simulink model "Threephaseplll"  (R2015b)
settings: Solver=VariableStepAuto  StartTime=0.0  StopTime=0.5  RelTol=1e-3
undefined symbols (not defined in the file): c, k, n, Ts, w1
libraries: powerlib_meascontrol x1, simulink x1, powerlib x1
settings Model: Creator=HP  LastModifiedBy=HP

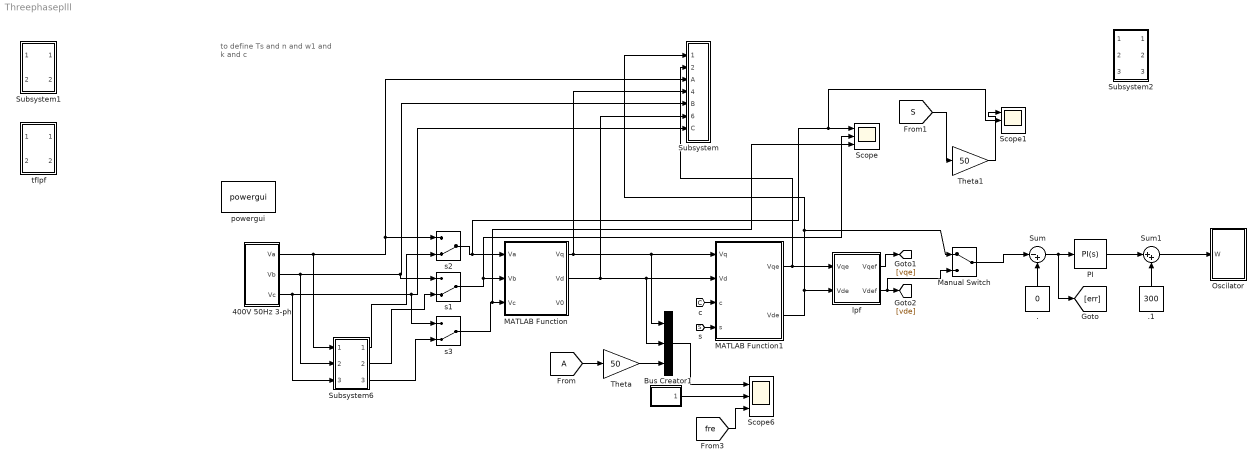
== system Threephaseplll ==
  note: to define Ts  and n
      | and w1 and k and c
  "               " : Subsystem
  . : Constant  Value=0
  .1 : Constant  Value=300
  400V 50Hz 3-ph : Subsystem
  Bus Creator1 : BusCreator  Inputs=3
  MATLAB Function : MATLAB Function  TreatAsAtomicUnit=on
  MATLAB Function1 : MATLAB Function  TreatAsAtomicUnit=on
  Manual Switch : ManualSwitch
  Oscilator : Subsystem
  PI : simulink/Continuous/PID Controller  Controller=PI  TimeDomain=Continuous-time  SampleTime=-1  IntegratorMethod=Forward Euler  FilterMethod=Forward Euler  Form=Parallel  UseFilter=on  ControllerParametersSource=internal  P=4  I=30  D=0  N=100  InitialConditionSource=internal  InitialConditionForIntegrator=0  InitialConditionForFilter=0  ExternalReset=none  ZeroCross=off  LimitOutput=off  UpperSaturationLimit=inf  LowerSaturationLimit=-inf  LinearizeAsGain=on  AntiWindupMode=none  Kb=1  TrackingMode=off  Kt=1  PParamMin=[]  PParamMax=[]  IParamMin=[]  IParamMax=[]  DParamMin=[]  DParamMax=[]  NParamMin=[]  NParamMax=[]  KbParamMin=[]  KbParamMax=[]  KtParamMin=[]  KtParamMax=[]  POutMin=[]  POutMax=[]  IOutMin=[]  IOutMax=[]  DOutMin=[]  DOutMax=[]  NOutMin=[]  NOutMax=[]  KbOutMin=[]  KbOutMax=[]  KtOutMin=[]  KtOutMax=[]  IntegratorOutMin=[]  IntegratorOutMax=[]  FilterOutMin=[]  FilterOutMax=[]  SumOutMin=[]  SumOutMax=[]  SumI1OutMin=[]  SumI1OutMax=[]  SumI2OutMin=[]  SumI2OutMax=[]  SumI3OutMin=[]  SumI3OutMax=[]  SumDOutMin=[]  SumDOutMax=[]  SaturationOutMin=[]  SaturationOutMax=[]  IntegratorContinuousStateAttributes=''  IntegratorStateMustResolveToSignalObject=off  IntegratorRTWStateStorageClass=Auto  FilterContinuousStateAttributes=''  FilterStateMustResolveToSignalObject=off  FilterRTWStateStorageClass=Auto  DifferentiatorICPrevScaledInput=0  DifferentiatorOutMin=[]  DifferentiatorOutMax=[]
  Scope : Scope  NumInputPorts=3
  Scope1 : Scope  NumInputPorts=3
  Scope6 : Scope  NumInputPorts=3
  Subsystem : Subsystem
  Subsystem1 : Subsystem
  Subsystem2 : Subsystem
  Subsystem6 : Subsystem
  Sum : Sum  Inputs=|-+
  Sum1 : Sum  Inputs=|++
  Theta : Gain  Gain=50
  Theta1 : Gain  Gain=50
  lpf : Subsystem
  powergui : powerlib/powergui  Priority=1  SimulationMode=Discrete  SolverType=Tustin/Backward Euler (TBE)  SampleTime=50e-6  frequency=60  SPID=on  DisableSnubberDevices=off  DisableRonSwitches=off  DisableVfSwitches=off  SwTol=0  DisplayEquations=on  Interpol=off  ExternalGateDelay=off  methode=off  Ts=10  FunctionMessages=off  echomessages=off  HookPort=off  EnableUseOfTLC=off  x0status=blocks  frequencyindice=50  Pbase=100e6  ErrMax=1e-4  Iterations=50  UnitsV=kV  UnitsW=MW  buscounter=0  RestoreLinks=warning  ResistiveCurrentMeasurement=off  Frange=[0:2:500]  Ylog=off  Xlog=on  ShowGrid=off  save=off  variable=ZData  structure=Vload  ZoomFFT=on  StartTime=0.2  cycles=4  DisplayStyle=3  fundamental=50  FreqAxis=on  MaxFrequency=1000  frequencyindicesteady=1  RmsSteady=1  display=off
  s1 : ManualSwitch  CurrentSetting=0
  s2 : ManualSwitch  CurrentSetting=0
  "s3 " : ManualSwitch  CurrentSetting=0
  tflpf : Subsystem
  wires:
  400V 50Hz 3-ph/1(Va) -> s2/1, Subsystem/3(A), Subsystem6/1(In1)
  400V 50Hz 3-ph/2(Vb) -> s1/1, Subsystem/5(B), Subsystem6/2(In2)
  400V 50Hz 3-ph/3(Vc) -> "s3 "/1, Subsystem/7(C), Subsystem6/3(In3)
  MATLAB Function/2(Vd) -> Subsystem/6("Vd "), MATLAB Function1/2(Vd), Bus Creator1/2
  Sum/1 -> [err], PI/1
  .1/1 -> Sum1/2
  MATLAB Function1/2(Vde) -> Manual Switch/1, Subsystem/1(Vde), lpf/2(Vde)
  ./1 -> Sum/2
  MATLAB Function/1(Vq) -> Subsystem/4(Vq), MATLAB Function1/1(Vq), Bus Creator1/1
  PI/1 -> Sum1/1
  MATLAB Function1/1(Vqe) -> Subsystem/2(Vqe), lpf/1(Vqe)
  Manual Switch/1 -> Sum/1
  lpf/2(Vdef) -> Manual Switch/2, [vde]
  [S] -> MATLAB Function1/4(s)
  [C] -> MATLAB Function1/3(c)
  lpf/1(Vqef) -> [vqe]
  Sum1/1 -> Oscilator/1(W)
  Theta/1 -> Bus Creator1/3
  [fre] -> Scope6/3
  Bus Creator1/1 -> Scope6/1
  [A] -> Theta/1
  "               "/1(Error PI) -> Scope6/2
  s2/1 -> Scope1/2, Scope/1, MATLAB Function/1(Va)
  s1/1 -> Scope/2, MATLAB Function/2(Vb)
  "s3 "/1 -> Scope/3, MATLAB Function/3(Vc)
  Subsystem6/1(Out1) -> s2/2
  Subsystem6/2(Out2) -> s1/2
  Subsystem6/3(Out3) -> "s3 "/2
  [S] -> Theta1/1
  Theta1/1 -> Scope1/1

== system Threephaseplll/                ==
  Error : Gain
  Error PI : Outport
  wires:
  Error/1 -> Error PI/1
  [err] -> Error/1

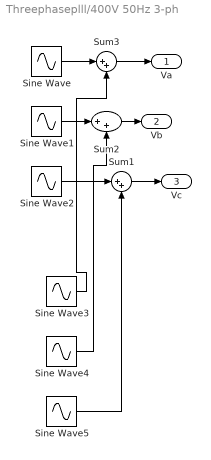
== system Threephaseplll/400V 50Hz 3-ph ==
  Sine Wave : Sin  Amplitude=c*400*sqrt(2)/sqrt(3)  Frequency=w1  SampleTime=Ts
  Sine Wave1 : Sin  Amplitude=400*sqrt(2)/sqrt(3)  Frequency=w1  Phase=-2*pi/3  SampleTime=Ts
  Sine Wave2 : Sin  Amplitude=400*sqrt(2)/sqrt(3)  Frequency=w1  Phase=-4*pi/3  SampleTime=Ts
  Sine Wave3 : Sin  Amplitude=0.2*400*sqrt(2)/sqrt(3)*k  Frequency=w1*n  SampleTime=Ts
  Sine Wave4 : Sin  Amplitude=0.2*k*400*sqrt(2)/sqrt(3)  Frequency=w1*n  Phase=-2*pi/3*n  SampleTime=Ts
  Sine Wave5 : Sin  Amplitude=0.2*k*400*sqrt(2)/sqrt(3)  Frequency=w1*n  Phase=-4*pi/3*n  SampleTime=Ts
  Sum1 : Sum  Inputs=|++
  Sum2 : Sum  Inputs=|++
  Sum3 : Sum  Inputs=|++
  Va : Outport
  Vb : Outport  Port=2
  Vc : Outport  Port=3
  wires:
  Sine Wave/1 -> Sum3/1
  Sum3/1 -> Va/1
  Sine Wave1/1 -> Sum2/1
  Sum2/1 -> Vb/1
  Sine Wave2/1 -> Sum1/1
  Sum1/1 -> Vc/1
  Sine Wave3/1 -> Sum3/2
  Sine Wave4/1 -> Sum2/2
  Sine Wave5/1 -> Sum1/2

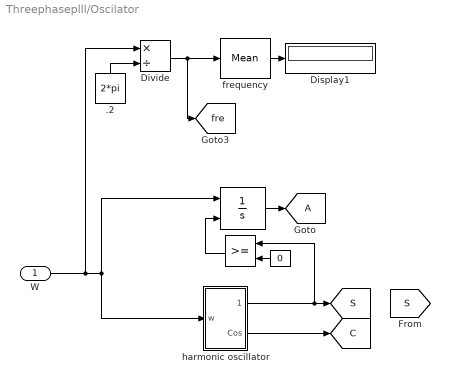
== system Threephaseplll/Oscilator ==
  W : Inport
  " " : Constant  Value=0
  "  " : Integrator  ExternalReset=rising  UpperSaturationLimit=2*pi  LowerSaturationLimit=0
  "    " : RelationalOperator  OutDataTypeStr=boolean
  .2 : Constant  Value=2*pi
  Display1 : Display
  Divide : Product  Inputs=*/
  frequency : powerlib_meascontrol/Measurements/Mean  Freq=60  Vinit=0  Ts=0
  "harmonic oscillator " : Subsystem
  tag scope: A=global, C=global, S=global, fre=global
  wires:
  .2/1 -> Divide/2
  "harmonic oscillator "/1(Sine) -> "    "/1, [S]
  "  "/1 -> [A]
  " "/1 -> "    "/2
  W/1 -> "harmonic oscillator "/1(w), "  "/1, Divide/1
  "    "/1 -> "  "/2
  frequency/1 -> Display1/1
  Divide/1 -> [fre], frequency/1
  "harmonic oscillator "/2(Cos) -> [C]

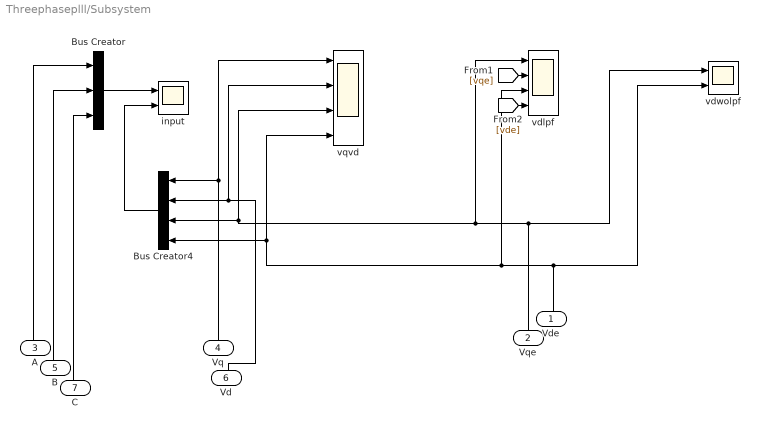
== system Threephaseplll/Subsystem ==
  Vde : Inport
  Vqe : Inport  Port=2
  A : Inport  Port=3
  Vq : Inport  Port=4
  B : Inport  Port=5
  "Vd " : Inport  Port=6
  C : Inport  Port=7
  Bus Creator : BusCreator  Inputs=3
  Bus Creator4 : BusCreator  Inputs=4
  input : Scope  NumInputPorts=2
  vdlpf : Scope  NumInputPorts=4
  vdwolpf : Scope  NumInputPorts=2
  vqvd : Scope  NumInputPorts=4
  wires:
  [vqe] -> vdlpf/2
  Bus Creator/1 -> input/1
  Bus Creator4/1 -> input/2
  "Vd "/1 -> vqvd/2, Bus Creator4/2
  A/1 -> Bus Creator/1
  B/1 -> Bus Creator/2
  Vq/1 -> vqvd/1, Bus Creator4/1
  Vqe/1 -> vdwolpf/1, vdlpf/1, vqvd/3, Bus Creator4/3
  C/1 -> Bus Creator/3
  Vde/1 -> vdwolpf/2, vdlpf/3, vqvd/4, Bus Creator4/4
  [vde] -> vdlpf/4

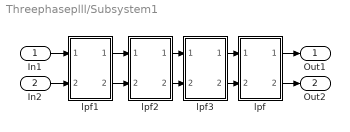
== system Threephaseplll/Subsystem1 ==
  In1 : Inport
  In2 : Inport  Port=2
  lpf : Subsystem
  lpf1 : Subsystem
  lpf2 : Subsystem
  lpf3 : Subsystem
  Out1 : Outport
  Out2 : Outport  Port=2
  wires:
  lpf1/2(Out2) -> lpf2/2(In2)
  lpf1/1(Out1) -> lpf2/1(In1)
  lpf2/2(Out2) -> lpf3/2(In2)
  lpf2/1(Out1) -> lpf3/1(In1)
  lpf3/1(Out1) -> lpf/1(In1)
  lpf3/2(Out2) -> lpf/2(In2)
  lpf/1(Out1) -> Out1/1
  lpf/2(Out2) -> Out2/1
  In2/1 -> lpf1/2(In2)
  In1/1 -> lpf1/1(In1)

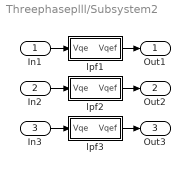
== system Threephaseplll/Subsystem2 ==
  In1 : Inport
  In2 : Inport  Port=2
  In3 : Inport  Port=3
  lpf1 : Subsystem
  lpf2 : Subsystem
  lpf3 : Subsystem
  Out1 : Outport
  Out2 : Outport  Port=2
  Out3 : Outport  Port=3
  wires:
  In2/1 -> lpf2/1(Vqe)
  In3/1 -> lpf3/1(Vqe)
  lpf2/1(Vqef) -> Out2/1
  lpf3/1(Vqef) -> Out3/1
  lpf1/1(Vqef) -> Out1/1
  In1/1 -> lpf1/1(Vqe)

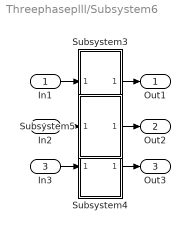
== system Threephaseplll/Subsystem6 ==
  In1 : Inport
  In2 : Inport  Port=2
  In3 : Inport  Port=3
  Subsystem3 : Subsystem
  Subsystem4 : Subsystem
  Subsystem5 : Subsystem
  Out1 : Outport
  Out2 : Outport  Port=2
  Out3 : Outport  Port=3
  wires:
  Subsystem5/1(Out1) -> Out2/1
  In1/1 -> Subsystem3/1(In1)
  Subsystem3/1(Out1) -> Out1/1
  Subsystem4/1(Out1) -> Out3/1
  In2/1 -> Subsystem5/1(In1)
  In3/1 -> Subsystem4/1(In1)

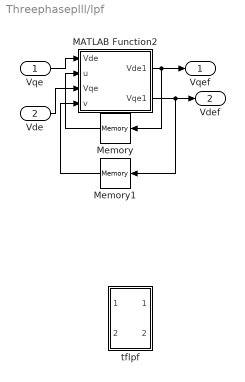
== system Threephaseplll/lpf ==
  Vqe : Inport
  Vde : Inport  Port=2
  MATLAB Function2 : MATLAB Function  TreatAsAtomicUnit=on
  Memory : Memory
  Memory1 : Memory
  tflpf : Subsystem
  Vqef : Outport
  Vdef : Outport  Port=2
  wires:
  MATLAB Function2/1(Vde1) -> Vqef/1, Memory/1
  Vqe/1 -> MATLAB Function2/1(Vde)
  Memory/1 -> MATLAB Function2/2(u)
  Vde/1 -> MATLAB Function2/3(Vqe)
  MATLAB Function2/2(Vqe1) -> Vdef/1, Memory1/1
  Memory1/1 -> MATLAB Function2/4(v)

== system Threephaseplll/tflpf ==
  In1 : Inport
  In2 : Inport  Port=2
  Transfer Fcn : TransferFcn  Numerator=[2*pi*10]  Denominator=[1 2*pi*10]
  Transfer Fcn1 : TransferFcn  Numerator=[2*pi*10]  Denominator=[1 2*pi*10]
  Out1 : Outport
  Out2 : Outport  Port=2
  wires:
  In2/1 -> Transfer Fcn1/1
  In1/1 -> Transfer Fcn/1
  Transfer Fcn/1 -> Out1/1
  Transfer Fcn1/1 -> Out2/1

== system Threephaseplll/Oscilator/harmonic oscillator  ==
  w : Inport
  MATLAB Function2 : MATLAB Function  TreatAsAtomicUnit=on
  Memory : Memory  X0=1
  Memory1 : Memory
  Sine : Outport
  Cos : Outport  Port=2
  wires:
  Memory1/1 -> MATLAB Function2/2(s)
  MATLAB Function2/2(s1) -> Sine/1, Memory1/1
  MATLAB Function2/1(c1) -> Cos/1, Memory/1
  Memory/1 -> MATLAB Function2/3(c)
  w/1 -> MATLAB Function2/1(u)

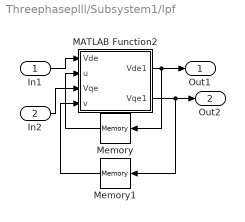
== system Threephaseplll/Subsystem1/lpf ==
  In1 : Inport
  In2 : Inport  Port=2
  MATLAB Function2 : MATLAB Function  TreatAsAtomicUnit=on
  Memory : Memory
  Memory1 : Memory
  Out1 : Outport
  Out2 : Outport  Port=2
  wires:
  MATLAB Function2/1(Vde1) -> Out1/1, Memory/1
  In1/1 -> MATLAB Function2/1(Vde)
  Memory/1 -> MATLAB Function2/2(u)
  In2/1 -> MATLAB Function2/3(Vqe)
  MATLAB Function2/2(Vqe1) -> Out2/1, Memory1/1
  Memory1/1 -> MATLAB Function2/4(v)

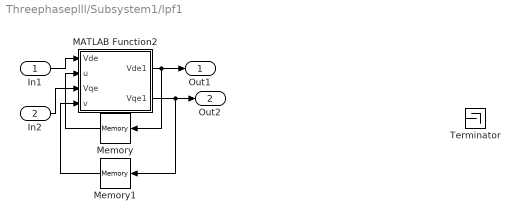
== system Threephaseplll/Subsystem1/lpf1 ==
  In1 : Inport
  In2 : Inport  Port=2
  MATLAB Function2 : MATLAB Function  TreatAsAtomicUnit=on
  Memory : Memory
  Memory1 : Memory
  Terminator : Terminator
  Out1 : Outport
  Out2 : Outport  Port=2
  wires:
  MATLAB Function2/1(Vde1) -> Out1/1, Memory/1
  In1/1 -> MATLAB Function2/1(Vde)
  Memory/1 -> MATLAB Function2/2(u)
  In2/1 -> MATLAB Function2/3(Vqe)
  MATLAB Function2/2(Vqe1) -> Out2/1, Memory1/1
  Memory1/1 -> MATLAB Function2/4(v)

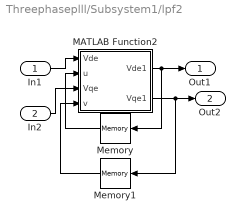
== system Threephaseplll/Subsystem1/lpf2 ==
  In1 : Inport
  In2 : Inport  Port=2
  MATLAB Function2 : MATLAB Function  TreatAsAtomicUnit=on
  Memory : Memory
  Memory1 : Memory
  Out1 : Outport
  Out2 : Outport  Port=2
  wires:
  MATLAB Function2/1(Vde1) -> Out1/1, Memory/1
  In1/1 -> MATLAB Function2/1(Vde)
  Memory/1 -> MATLAB Function2/2(u)
  In2/1 -> MATLAB Function2/3(Vqe)
  MATLAB Function2/2(Vqe1) -> Out2/1, Memory1/1
  Memory1/1 -> MATLAB Function2/4(v)

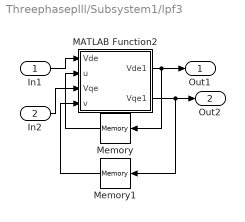
== system Threephaseplll/Subsystem1/lpf3 ==
  In1 : Inport
  In2 : Inport  Port=2
  MATLAB Function2 : MATLAB Function  TreatAsAtomicUnit=on
  Memory : Memory
  Memory1 : Memory
  Out1 : Outport
  Out2 : Outport  Port=2
  wires:
  MATLAB Function2/1(Vde1) -> Out1/1, Memory/1
  In1/1 -> MATLAB Function2/1(Vde)
  Memory/1 -> MATLAB Function2/2(u)
  In2/1 -> MATLAB Function2/3(Vqe)
  MATLAB Function2/2(Vqe1) -> Out2/1, Memory1/1
  Memory1/1 -> MATLAB Function2/4(v)

== system Threephaseplll/Subsystem2/lpf1 ==
  Vqe : Inport
  MATLAB Function2 : MATLAB Function  TreatAsAtomicUnit=on
  Memory : Memory
  Memory1 : Memory
  Vqef : Outport
  wires:
  MATLAB Function2/1(Vde1) -> Vqef/1, Memory/1
  Vqe/1 -> MATLAB Function2/1(Vde)
  Memory/1 -> MATLAB Function2/2(u)
  ? -> MATLAB Function2/3(Vqe)
  MATLAB Function2/2(Vqe1) -> Memory1/1
  Memory1/1 -> MATLAB Function2/4(v)

== system Threephaseplll/Subsystem2/lpf2 ==
  Vqe : Inport
  MATLAB Function2 : MATLAB Function  TreatAsAtomicUnit=on
  Memory : Memory
  Memory1 : Memory
  Vqef : Outport
  wires:
  MATLAB Function2/1(Vde1) -> Vqef/1, Memory/1
  Vqe/1 -> MATLAB Function2/1(Vde)
  Memory/1 -> MATLAB Function2/2(u)
  ? -> MATLAB Function2/3(Vqe)
  MATLAB Function2/2(Vqe1) -> Memory1/1
  Memory1/1 -> MATLAB Function2/4(v)

== system Threephaseplll/Subsystem2/lpf3 ==
  Vqe : Inport
  MATLAB Function2 : MATLAB Function  TreatAsAtomicUnit=on
  Memory : Memory
  Memory1 : Memory
  Vqef : Outport
  wires:
  MATLAB Function2/1(Vde1) -> Vqef/1, Memory/1
  Vqe/1 -> MATLAB Function2/1(Vde)
  Memory/1 -> MATLAB Function2/2(u)
  ? -> MATLAB Function2/3(Vqe)
  MATLAB Function2/2(Vqe1) -> Memory1/1
  Memory1/1 -> MATLAB Function2/4(v)

== system Threephaseplll/Subsystem6/Subsystem3 ==
  In1 : Inport
  Transfer Fcn{,1..3} (4 alike) : TransferFcn  Denominator=[(1/(2*pi*60)) 1]
  Out1 : Outport
  wires:
  Transfer Fcn1/1 -> Out1/1
  In1/1 -> Transfer Fcn/1
  Transfer Fcn3/1 -> Transfer Fcn1/1
  Transfer Fcn/1 -> Transfer Fcn2/1
  Transfer Fcn2/1 -> Transfer Fcn3/1

== system Threephaseplll/Subsystem6/Subsystem4 ==
  In1 : Inport
  Transfer Fcn{,1..3} (4 alike) : TransferFcn  Denominator=[(1/(2*pi*60)) 1]
  Out1 : Outport
  wires:
  Transfer Fcn1/1 -> Out1/1
  In1/1 -> Transfer Fcn/1
  Transfer Fcn3/1 -> Transfer Fcn1/1
  Transfer Fcn/1 -> Transfer Fcn2/1
  Transfer Fcn2/1 -> Transfer Fcn3/1

== system Threephaseplll/Subsystem6/Subsystem5 ==
  In1 : Inport
  Transfer Fcn{,1..3} (4 alike) : TransferFcn  Denominator=[(1/(2*pi*60)) 1]
  Out1 : Outport
  wires:
  Transfer Fcn1/1 -> Out1/1
  In1/1 -> Transfer Fcn/1
  Transfer Fcn3/1 -> Transfer Fcn1/1
  Transfer Fcn/1 -> Transfer Fcn2/1
  Transfer Fcn2/1 -> Transfer Fcn3/1

== system Threephaseplll/lpf/tflpf ==
  In1 : Inport
  In2 : Inport  Port=2
  Transfer Fcn : TransferFcn  Numerator=[2*pi*10]  Denominator=[1 2*pi*10]
  Transfer Fcn1 : TransferFcn  Numerator=[2*pi*10]  Denominator=[1 2*pi*10]
  Out1 : Outport
  Out2 : Outport  Port=2
  wires:
  In2/1 -> Transfer Fcn1/1
  In1/1 -> Transfer Fcn/1
  Transfer Fcn/1 -> Out1/1
  Transfer Fcn1/1 -> Out2/1

== matlab function Threephaseplll/MATLAB Function1 ==
  data: Vq input; Vqe output; Vd input; c input; s input; Vde output
function [Vqe,Vde] = fcn(Vq,Vd,c,s)
%#rotating frame transfer

Vqe=Vd*c+Vq*s;
Vde=Vd*s-Vq*c;
end

== matlab function Threephaseplll/MATLAB Function ==
  data: Va input; Vq output; Vb input; Vc input; Vd output; V0 output
function [Vq,Vd,V0] = fcn(Va,Vb,Vc)
%#transformation to other frame
x=2*pi/3;
%k=[1 cos(-x) cos(x);0 sin(-x) sin(x);0.5 0.5 0.5];
Vq=(2/3)*(Va+Vb*cos(-x)+Vc*cos(x));
Vd=(2/3)*(Vb*sin(-x)+Vc*sin(x));
%V3ph=[Va Vb Vc];
%V=k*V3ph;

V0=(1/3)*(Va+Vb+Vc);
end

== matlab function Threephaseplll/Oscilator/harmonic oscillator /MATLAB Function2 ==
  data: u input; s input; c input; c1 output; s1 output
function [c1,s1] = fcn(u,s,c)

Ts=5e-5;

    s1=s+u*Ts*c;
    
    c1=c-u*Ts*s1;
    if c1>1
        s1=0;
        c1=1;

    end
        
    
%     i1=i+0.001;
%     if >0.42
%        i=0;i1=0;
%         c1=1;
%         s1=0;
%     end

== matlab function Threephaseplll/lpf/MATLAB Function2 ==
  data: Vde input; Vde1 output; u input; Vqe input; v input; Vqe1 output
function [Vde1,Vqe1] = fcn(Vde,u,Vqe,v)
%#codegen
Ts=5e-5;
a=Ts/0.009;
%Vde1=u*a/(a+1)+(1/(1+a))*(Vde-u);
%Vqe1=v*a/(a+1)+(1/(1+a))*(Vqe-v);
Vde1=u+a*(Vde-u);
Vqe1=v+a*(Vqe-v);
end

== matlab function Threephaseplll/Subsystem1/lpf/MATLAB Function2 ==
  data: Vde input; Vde1 output; u input; Vqe input; v input; Vqe1 output
function [Vde1,Vqe1] = fcn(Vde,u,Vqe,v)
%#codegen
Ts=5e-5;
a=Ts/0.009;
%Vde1=u*a/(a+1)+(1/(1+a))*(Vde-u);
%Vqe1=v*a/(a+1)+(1/(1+a))*(Vqe-v);
Vde1=u+a*(Vde-u);
Vqe1=v+a*(Vqe-v);
end

== matlab function Threephaseplll/Subsystem1/lpf1/MATLAB Function2 ==
  data: Vde input; Vde1 output; u input; Vqe input; v input; Vqe1 output
function [Vde1,Vqe1] = fcn(Vde,u,Vqe,v)
%#codegen
Ts=5e-5;
a=Ts/0.009;
%Vde1=u*a/(a+1)+(1/(1+a))*(Vde-u);
%Vqe1=v*a/(a+1)+(1/(1+a))*(Vqe-v);
Vde1=u+a*(Vde-u);
Vqe1=v+a*(Vqe-v);
end

== matlab function Threephaseplll/Subsystem1/lpf2/MATLAB Function2 ==
  data: Vde input; Vde1 output; u input; Vqe input; v input; Vqe1 output
function [Vde1,Vqe1] = fcn(Vde,u,Vqe,v)
%#codegen
Ts=5e-5;
a=Ts/0.009;
%Vde1=u*a/(a+1)+(1/(1+a))*(Vde-u);
%Vqe1=v*a/(a+1)+(1/(1+a))*(Vqe-v);
Vde1=u+a*(Vde-u);
Vqe1=v+a*(Vqe-v);
end

== matlab function Threephaseplll/Subsystem1/lpf3/MATLAB Function2 ==
  data: Vde input; Vde1 output; u input; Vqe input; v input; Vqe1 output
function [Vde1,Vqe1] = fcn(Vde,u,Vqe,v)
%#codegen
Ts=5e-5;
a=Ts/0.009;
%Vde1=u*a/(a+1)+(1/(1+a))*(Vde-u);
%Vqe1=v*a/(a+1)+(1/(1+a))*(Vqe-v);
Vde1=u+a*(Vde-u);
Vqe1=v+a*(Vqe-v);
end

== matlab function Threephaseplll/Subsystem2/lpf1/MATLAB Function2 ==
  data: Vde input; Vde1 output; u input; Vqe input; v input; Vqe1 output
function [Vde1,Vqe1] = fcn(Vde,u,Vqe,v)
%#codegen
Ts=5e-5;
f=60;
a=Ts*2*pi*f;
%Vde1=u*a/(a+1)+(1/(1+a))*(Vde-u);
%Vqe1=v*a/(a+1)+(1/(1+a))*(Vqe-v);
Vde1=u+a*(Vde-u);
Vqe1=v+a*(Vqe-v);
end

== matlab function Threephaseplll/Subsystem2/lpf2/MATLAB Function2 ==
  data: Vde input; Vde1 output; u input; Vqe input; v input; Vqe1 output
function [Vde1,Vqe1] = fcn(Vde,u,Vqe,v)
%#codegen
Ts=5e-5;
f=60;
a=Ts*2*pi*f;
%Vde1=u*a/(a+1)+(1/(1+a))*(Vde-u);
%Vqe1=v*a/(a+1)+(1/(1+a))*(Vqe-v);
Vde1=u+a*(Vde-u);
Vqe1=v+a*(Vqe-v);
end

== matlab function Threephaseplll/Subsystem2/lpf3/MATLAB Function2 ==
  data: Vde input; Vde1 output; u input; Vqe input; v input; Vqe1 output
function [Vde1,Vqe1] = fcn(Vde,u,Vqe,v)
%#codegen
Ts=5e-5;
f=60;
a=Ts*2*pi*f;
%Vde1=u*a/(a+1)+(1/(1+a))*(Vde-u);
%Vqe1=v*a/(a+1)+(1/(1+a))*(Vqe-v);
Vde1=u+a*(Vde-u);
Vqe1=v+a*(Vqe-v);
end
